simulink model "AM_v2"  (R2020b)
settings: Solver=ode45  StartTime=0.0  StopTime=10.0  RelTol=1e-3
libraries: dsparch4 x2, commchan3 x1
settings Model: Creator=xiao'xin  LastModifiedBy=xiao'xin
settings DataIOCC: LimitDataPoints=on  SaveFormat=Array  ReturnWorkspaceOutputs=off
settings OptimizationCC: BlockReduction=off  BooleanDataType=off  LifeSpan=inf
settings DebuggingCC: SaveWithParameterizedLinksMsg=none  UnderspecifiedInitializationDetection=Classic  MergeDetectMultiDrivingBlocksExec=none  SignalResolutionControl=TryResolveAllWithWarning  SFUnexpectedBacktrackingDiag=warning  SFNoUnconditionalDefaultTransitionDiag=warning  SFExecutionAtInitializationDiag=none  ArithmeticOperatorsInVariantConditions=warning
settings HardwareCC: ProdBitPerPointer=32  ProdBitPerSizeT=32  ProdBitPerPtrDiffT=32  ProdLargestAtomicFloat=None  ProdIntDivRoundTo=Undefined  ProdEndianess=Unspecified  ProdWordSize=32  ProdHWDeviceType=32-bit Generic  TargetUnknown=on
settings ModelReferenceCC: PropagateSignalLabelsOutOfModel=off
settings SFSimCC: SimUseLocalCustomCode=off  CustomCodeUndefinedFunction=UseInterfaceOnly
settings RTWCC: RTWUseLocalCustomCode=off
settings CodeAppCC: StateflowObjectComments=on
settings GRTTargetCC: TargetLangStandard=C89/C90 (ANSI)
settings ConfigComp: CovMetricSettings=dw  CovSaveCumulativeToWorkspaceVar=on  CovSaveSingleToWorkspaceVar=on  CovExternalEMLEnable=off  CovSFcnEnable=off

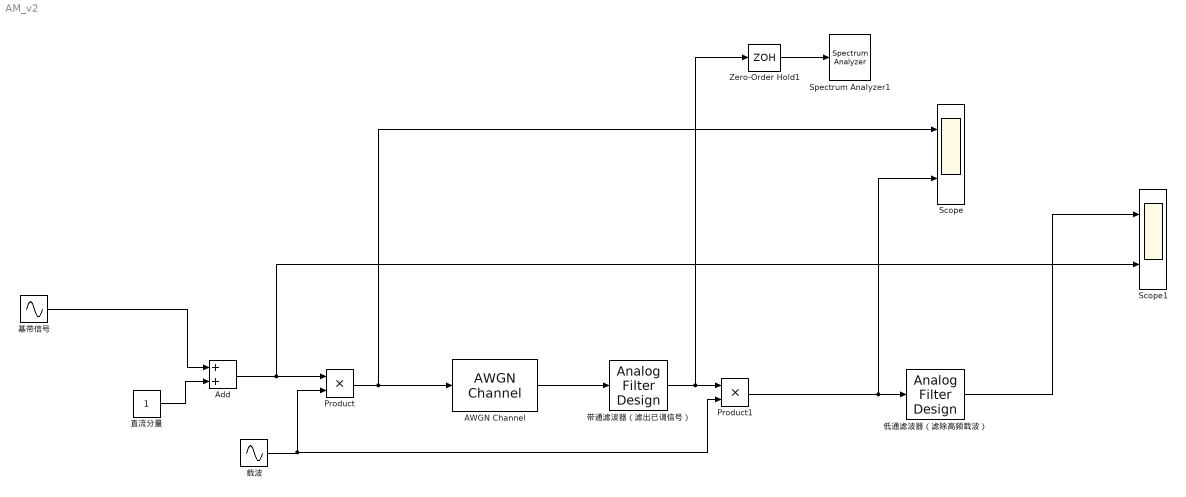
== system AM_v2 ==
  AWGN Channel : commchan3/AWGN Channel  InputProcessing=Columns as channels (frame based)  seed=67  noiseMode="Signal to noise ratio  (SNR)"  EbNodB=10  EsNodB=10  SNRdB=20  bitsPerSym=1  Ps=1  Tsym=1  variance=1
  Add : Sum
  Product : Product
  Product1 : Product
  Scope : Scope  NumInputPorts=2
  Scope1 : Scope  NumInputPorts=2
  Spectrum Analyzer1 : SpectrumAnalyzer
  Zero-Order Hold1 : ZeroOrderHold  SampleTime=0.00001
  低通滤波器（滤除高频载波） : dsparch4/Analog Filter Design  method=Butterworth  filttype=Lowpass  N=8  Wlo=1000*2*pi  Whi=80  Rp=2  Rs=40
  基带信号 : Sin  Frequency=300*2*pi  SampleTime=0
  带通滤波器（滤出已调信号） : dsparch4/Analog Filter Design  method=Butterworth  filttype=Bandpass  N=8  Wlo=9500*2*pi  Whi=10500*2*pi  Rp=2  Rs=40
  直流分量 : Constant
  载波 : Sin  Amplitude=5  Frequency=10000*2*pi  SampleTime=0
  wires:
  基带信号/1 -> Add/1
  直流分量/1 -> Add/2
  Add/1 -> Scope1/2, Product/1
  载波/1 -> Product1/2, Product/2
  AWGN Channel/1 -> 带通滤波器（滤出已调信号）/1
  带通滤波器（滤出已调信号）/1 -> Zero-Order Hold1/1, Product1/1
  Product1/1 -> 低通滤波器（滤除高频载波）/1, Scope/2
  低通滤波器（滤除高频载波）/1 -> Scope1/1
  Zero-Order Hold1/1 -> Spectrum Analyzer1/1
  Product/1 -> AWGN Channel/1, Scope/1
